simulink model "PMSM_2017b_WithRslvr"  (R2017b)
settings: Solver=FixedStepDiscrete  StartTime=0.0  StopTime=0.2  FixedStep=Ts  RelTol=1e-4  EnableMultiTasking=on
values from neighbouring files (symbols this model uses):
  Ba = 0    [initialization.m]
  Fl = 0.007    [initialization.m]
  flux = Kt/(1.5*P*sqrt(2))    [initialization.m]
  fpwm = 1e4    (= 10000)    [initialization.m]
  Imax = 6*sqrt(2)    [initialization.m]
  J = 9.96e-5    (= 9.96e-05)    [initialization.m]
  K1 = wn^2    (= 1000000)    [initialization.m]
  K2 = 2*fei/wn    (= 0.002)    [initialization.m]
  K_resolver = 1    [initialization.m]
  Ki_Cctrl_d = Rs/(4*Tpwm)    (= 22125)    [initialization.m]
  Ki_Cctrl_q = parameters(4)    [cal_n.m]    (also in draw.m; draw_n_I.m; initialization.m = 1)
  Ki_Spdctrl = parameters(2)    [cal_n.m]    (also in draw.m; draw_n_I.m; initialization.m = 1)
  Kp_Cctrl_d = Ld/(4*Tpwm)    (= 462.5)    [initialization.m]
  Kp_Cctrl_q = parameters(3)    [cal_n.m]    (also in draw.m; draw_n_I.m; initialization.m = 1)
  Kp_Spdctrl = parameters(1)    [cal_n.m]    (also in draw.m; draw_n_I.m; initialization.m = 1)
  Kt = 1.32    [initialization.m]
  Ld = 0.185    [initialization.m]
  Lq = 0.185    [initialization.m]
  P = X    [PSO.m]    (also in initialization.m = 2)
  Rs = 17.7/2    (= 8.85)    [initialization.m]
  SinPeakValue = 0.95104    [initialization.m]
  TestCurrentController = 0    [initialization.m]
  Tf = 0.08    [initialization.m]
  Tpwm = 1e-4    (= 0.0001)    [initialization.m]
  Ts = 1e-5    (= 1e-05)    [initialization.m]
  Udc = 230    [initialization.m]
  UseAgAtan2 = 0    [initialization.m]
  UseAgSim = 1    [initialization.m]
  wm_base = 3000*pi/30    (= 314.159265359)    [initialization.m]
undefined symbols (not defined in the file or in its folder): DiscIntNeverNeededParam
libraries: powerlib x6, simulink x5, dspmtrx3 x1
settings Model: Creator=SUN  LastModifiedBy=Administrator
settings SolverCC: ZeroCrossControl=DisableAll
settings DataIOCC: LimitDataPoints=on  SaveFormat=Array  SignalLoggingSaveFormat=ModelDataLogs
settings OptimizationCC: ExpressionDepthLimit=2147483647  InitFltsAndDblsToZero=on  LifeSpan=inf
settings DebuggingCC: UnderspecifiedInitializationDetection=Classic  MergeDetectMultiDrivingBlocksExec=none  SolverPrmCheckMsg=warning  FcnCallInpInsideContextMsg=warning  StateNameClashWarn=warning  SFUnexpectedBacktrackingDiag=warning  SFNoUnconditionalDefaultTransitionDiag=warning  SFExecutionAtInitializationDiag=none
settings HardwareCC: ProdBitPerPointer=32  ProdBitPerSizeT=32  ProdBitPerPtrDiffT=32  ProdLargestAtomicFloat=None  ProdIntDivRoundTo=Undefined  ProdEndianess=Unspecified  ProdWordSize=32  ProdHWDeviceType=32-bit Generic
settings ModelReferenceCC: PropagateSignalLabelsOutOfModel=off
settings CodeAppCC: StateflowObjectComments=on
settings GRTTargetCC: TargetLangStandard=C89/C90 (ANSI)  GeneratePreprocessorConditionals=Disable all  CombineOutputUpdateFcns=off  GRTInterface=on
settings ConfigComp: CovMetricSettings=dw  CovHtmlReporting=on  CovSaveCumulativeToWorkspaceVar=on  CovSaveSingleToWorkspaceVar=on  CovExternalEMLEnable=off
settings SimscapeCC: SimscapeNormalizeSystem=off

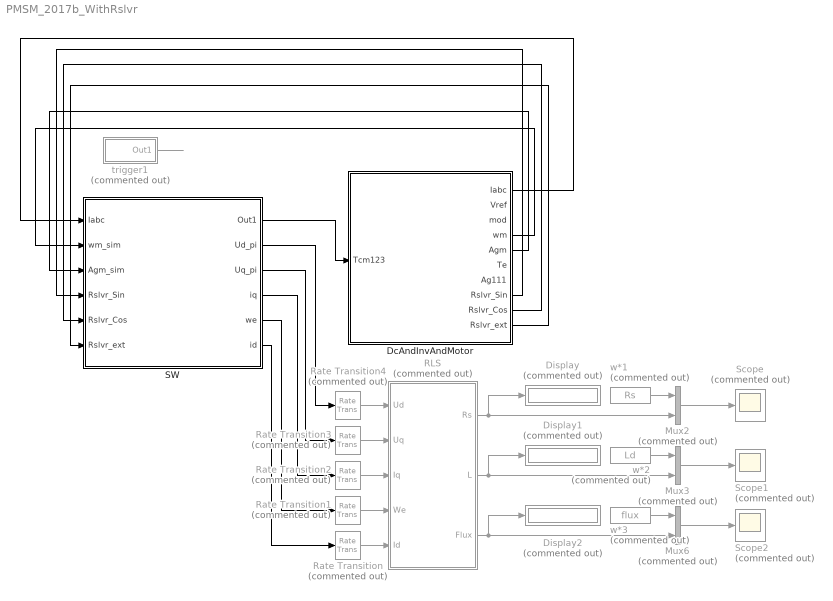
== system PMSM_2017b_WithRslvr ==
  DcAndInvAndMotor : Subsystem
  Display : Display  Commented=on
  Display1 : Display  Commented=on
  Display2 : Display  Commented=on
  Mux2 : Mux  Commented=on  Inputs=2
  Mux3 : Mux  Commented=on  Inputs=2
  Mux6 : Mux  Commented=on  Inputs=2
  RLS : Subsystem  Commented=on
      mask Display: disp('RLS');
  Rate Transition{,1..4} (5 alike) : RateTransition  Commented=on
  SW : Subsystem
  Scope : Scope  Commented=on
  Scope1 : Scope  Commented=on
  Scope2 : Scope  Commented=on
  trigger1 : Subsystem  Commented=on
  w*1 : Constant  Commented=on  Value=Rs
  w*2 : Constant  Commented=on  Value=Ld
  w*3 : Constant  Commented=on  Value=flux
  wires:
  w*3/1 -> Mux6/1
  Mux6/1 -> Scope2/1
  RLS/3(Flux) -> Display2/1, Mux6/2
  w*2/1 -> Mux3/1
  Mux3/1 -> Scope1/1
  w*1/1 -> Mux2/1
  RLS/1(Rs) -> Mux2/2, Display/1
  Mux2/1 -> Scope/1
  RLS/2(L) -> Display1/1, Mux3/2
  trigger1/1(Out1) -> ?
  SW/1(Out1) -> DcAndInvAndMotor/1(Tcm123)
  DcAndInvAndMotor/1(Iabc) -> SW/1(Iabc)
  SW/4(iq) -> Rate Transition2/1
  SW/5(we) -> Rate Transition1/1
  SW/2(Ud_pi) -> Rate Transition4/1
  SW/3(Uq_pi) -> Rate Transition3/1
  SW/6(id) -> Rate Transition/1
  Rate Transition/1 -> RLS/5(Id)
  Rate Transition1/1 -> RLS/4(We)
  Rate Transition2/1 -> RLS/3(Iq)
  Rate Transition3/1 -> RLS/2(Uq)
  Rate Transition4/1 -> RLS/1(Ud)
  DcAndInvAndMotor/5(Agm) -> SW/3(Agm_sim)
  DcAndInvAndMotor/8(Rslvr_Sin) -> SW/4(Rslvr_Sin)
  DcAndInvAndMotor/9(Rslvr_Cos) -> SW/5(Rslvr_Cos)
  DcAndInvAndMotor/10(Rslvr_ext) -> SW/6(Rslvr_ext)
  DcAndInvAndMotor/4(wm) -> SW/2(wm_sim)

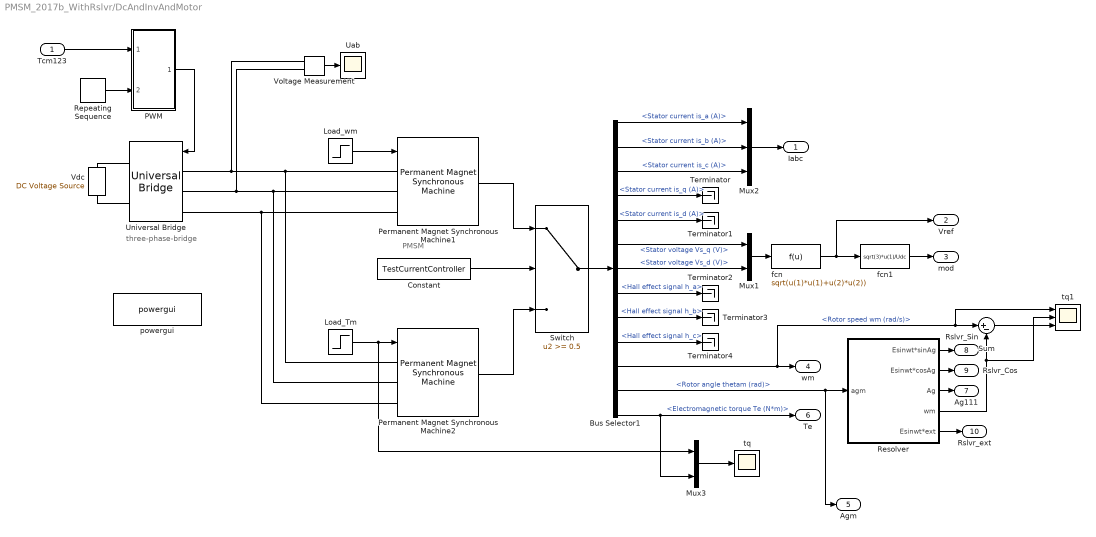
== system PMSM_2017b_WithRslvr/DcAndInvAndMotor ==
  note: three-phase-bridge
  note: PMSM
  Tcm123 : Inport
  Bus Selector1 : BusSelector  OutputSignals=Stator current is_a (A),Stator current is_b (A),Stator current is_c (A),Stator current is_q (A),Stator current is_d (A),Stator voltage Vs_q (V),Stator voltage Vs_d (V),Hall effect signal h_a,Hall effect signal h_b,Hall effect signal h_c,Rotor speed wm (rad/s),Rotor angle thetam (rad),Electromagnetic torque Te (N*m)
  Constant : Constant  Value=TestCurrentController
  Load_Tm : Step  Time=0.15  After=0  SampleTime=0
  Load_wm : Step  Time=0.15  Before=30  After=100  SampleTime=0
  Mux1 : Mux  Inputs=2
  Mux2 : Mux  Inputs=3
  Mux3 : Mux  Inputs=2
  PWM : Subsystem
  Permanent Magnet Synchronous Machine1 : powerlib/Machines/Permanent Magnet Synchronous Machine  NbPhases=3  FluxDistribution=Sinusoidal  RotorType=Salient-pole  MechanicalLoad=Speed w  PresetModel=No  ShowDetailedParameters=on  MeasurementBus=off  Resistance=Rs  Inductance=8.5e-3  dqInductances=[Ld Lq]  La=Lq  MachineConstant=Flux linkage established by magnets (V.s)  Flux=flux  VoltageCst=112.8644  TorqueCst=0.93338  Flat=120  Mechanical=[J Fl P Tf]  PolePairs=P  InitialConditions=[0,0,0,0]  InitialConditions5ph=[0 0 0 0 0 0]  TsPowergui=0  TsBlock=-1  RefAngle=Aligned with phase A axis (original Park)
      settings: SourceProductName=Simscape Power Systems
  Permanent Magnet Synchronous Machine2 : powerlib/Machines/Permanent Magnet Synchronous Machine  NbPhases=3  FluxDistribution=Sinusoidal  RotorType=Salient-pole  MechanicalLoad=Torque Tm  PresetModel=No  ShowDetailedParameters=on  MeasurementBus=off  Resistance=Rs  Inductance=8.5e-3  dqInductances=[Ld Lq]  La=Lq  MachineConstant=Flux linkage established by magnets (V.s)  Flux=flux  VoltageCst=112.8644  TorqueCst=0.93338  Flat=120  Mechanical=[J Fl P Tf]  PolePairs=P  InitialConditions=[0,0,0,0]  InitialConditions5ph=[0 0 0 0 0 0]  TsPowergui=0  TsBlock=-1  RefAngle=Aligned with phase A axis (original Park)
      settings: SourceProductName=Simscape Power Systems
  Repeating Sequence : simulink/Sources/Repeating Sequence  rep_seq_t=[0 Tpwm/2 Tpwm]  rep_seq_y=[0 Tpwm/2 0]
  Resolver : Subsystem
  Sum : Sum  Inputs=|+-
  Switch : Switch  Threshold=0.5
  Terminator{,1..4} (5 alike) : Terminator
  Uab : Scope
  Universal Bridge : powerlib/Power Electronics/Universal Bridge  Arms=3  SnubberResistance=1e5  SnubberCapacitance=inf  Device=IGBT / Diodes  Ron=1e-3  Lon=0  ForwardVoltages="[  0  0  ]"  ForwardVoltage=0  GTOparameters=[ 10e-6 , 20e-6 ]  IGBTparameters=[ 1e-6 , 2e-6 ]  Measurements=None  Measurements_2=None  converterType=Rectifier
  Vdc : powerlib/Electrical Sources/DC Voltage Source  Amplitude=Udc  Measurements=Voltage
  Voltage Measurement : powerlib/Measurements/Voltage Measurement  PhasorSimulation=off  OutputType=Complex  PSBequivalent=0
  fcn : Fcn  Expr=sqrt(u(1)*u(1)+u(2)*u(2))
  fcn1 : Fcn  Expr=sqrt(3)*u(1)/Udc
  powergui : powerlib/powergui  SimulationMode=Discrete  SampleTime=Ts  frequency=60  Iterations=50  frequencyindice=0  Pbase=100e6  ErrMax=1e-4  UnitsV=kV  UnitsW=MW  buscounter=0  FunctionMessages=off  echomessages=off  EnableUseOfTLC=off  CurrentSourceSwitches=off  DisableSnubberDevices=off  DisableRonSwitches=off  DisableVfSwitches=off  DisplayEquations=off  SolverType=Backward Euler  Interpol=off  ExternalGateDelay=off  methode=off  Ts=0  x0status=blocks  SPID=off  SwTol=0  HookPort=off  RestoreLinks=warning  ResistiveCurrentMeasurement=off  Frange=[0:2:500]  Ylog=off  Xlog=on  ShowGrid=off  save=off  variable=ZData  structure=0  ZoomFFT=on  StartTime=0.0  cycles=1  DisplayStyle=1  fundamental=60  FreqAxis=off  MaxFrequency=1000  frequencyindicesteady=1  RmsSteady=1  display=off
  tq : Scope
  tq1 : Scope  NumInputPorts=3
  Iabc : Outport
  Vref : Outport  Port=2
  mod : Outport  Port=3
  wm : Outport  Port=4
  Agm : Outport  Port=5
  Te : Outport  Port=6
  Ag111 : Outport  Port=7
  Rslvr_Sin : Outport  Port=8
  Rslvr_Cos : Outport  Port=9
  Rslvr_ext : Outport  Port=10
  wires:
  Voltage Measurement/1 -> Uab/1
  Mux1/1 -> fcn/1
  fcn1/1 -> mod/1
  fcn/1 -> Vref/1, fcn1/1
  Bus Selector1/1 -> Mux2/1  "<Stator current is_a (A)>"
  Bus Selector1/2 -> Mux2/2  "<Stator current is_b (A)>"
  Bus Selector1/3 -> Mux2/3  "<Stator current is_c (A)>"
  Mux2/1 -> Iabc/1
  Bus Selector1/6 -> Mux1/1  "<Stator voltage Vs_q (V)>"
  Bus Selector1/7 -> Mux1/2  "<Stator voltage Vs_d (V)>"
  Bus Selector1/13 -> Mux3/2, Te/1  "<Electromagnetic torque Te (N*m)>"
  Bus Selector1/11 -> tq1/1, Sum/1, wm/1  "<Rotor speed wm (rad/s)>"
  Bus Selector1/4 -> Terminator/1  "<Stator current is_q (A)>"
  Bus Selector1/5 -> Terminator1/1  "<Stator current is_d (A)>"
  Bus Selector1/8 -> Terminator2/1  "<Hall effect signal h_a>"
  Bus Selector1/9 -> Terminator3/1  "<Hall effect signal h_b>"
  Bus Selector1/10 -> Terminator4/1  "<Hall effect signal h_c>"
  Permanent Magnet Synchronous Machine1/1 -> Switch/1
  Permanent Magnet Synchronous Machine2/1 -> Switch/3
  Switch/1 -> Bus Selector1/1
  Constant/1 -> Switch/2
  Load_wm/1 -> Permanent Magnet Synchronous Machine1/1
  Load_Tm/1 -> Mux3/1, Permanent Magnet Synchronous Machine2/1
  Mux3/1 -> tq/1
  PWM/1(PWM) -> Universal Bridge/1
  Repeating Sequence/1 -> PWM/2(Carrier)
  Tcm123/1 -> PWM/1(Tcm123)
  Bus Selector1/12 -> Agm/1, Resolver/1(agm)  "<Rotor angle thetam (rad)>"
  Resolver/4(wm) -> tq1/2, Sum/2
  Resolver/3(Ag) -> Ag111/1
  Sum/1 -> tq1/3
  Resolver/2(Esinwt*cosAg) -> Rslvr_Cos/1
  Resolver/1(Esinwt*sinAg) -> Rslvr_Sin/1
  Resolver/5(Esinwt*ext) -> Rslvr_ext/1
  connections:
  Universal Bridge/RConn1 -- Vdc/RConn1
  Universal Bridge/RConn2 -- Vdc/LConn1
  Permanent Magnet Synchronous Machine1/LConn1 -- Permanent Magnet Synchronous Machine2/LConn1 -- Voltage Measurement/LConn1 -- Universal Bridge/LConn1
  Permanent Magnet Synchronous Machine1/LConn2 -- Permanent Magnet Synchronous Machine2/LConn2 -- Voltage Measurement/LConn2 -- Universal Bridge/LConn2
  Permanent Magnet Synchronous Machine1/LConn3 -- Permanent Magnet Synchronous Machine2/LConn3 -- Universal Bridge/LConn3

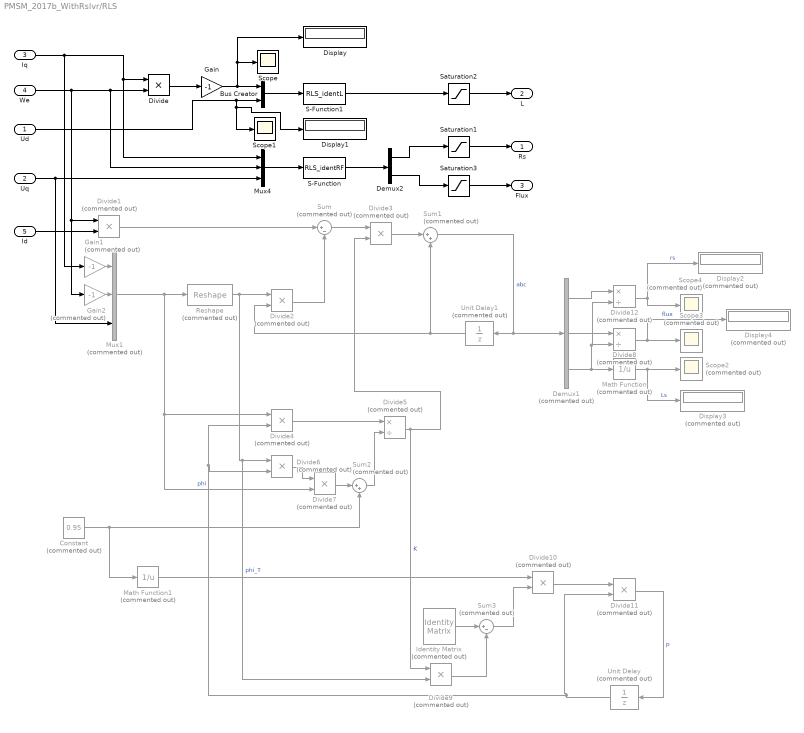
== system PMSM_2017b_WithRslvr/RLS ==
  Ud : Inport
  Uq : Inport  Port=2
  Iq : Inport  Port=3
  We : Inport  Port=4
  Id : Inport  Port=5
  Bus Creator : BusCreator  Inputs=2
  Constant : Constant  Commented=on  Value=0.95
  Demux1 : Demux  Commented=on  Outputs=3
  Demux2 : Demux  Outputs=2
  Display : Display
  Display1 : Display
  Display2 : Display  Commented=on
  Display3 : Display  Commented=on
  Display4 : Display  Commented=on
  Divide : Product  Inputs=**
  Divide{1..4,6..7,9..11} (9 alike) : Product  Commented=on  Inputs=**
  Divide12 : Product  Commented=on  Inputs=*/
  Divide5 : Product  Commented=on  Inputs=*/
  Divide8 : Product  Commented=on  Inputs=*/
  Gain : Gain  Gain=-1
  Gain1 : Gain  Commented=on  Gain=-1
  Gain2 : Gain  Commented=on  Gain=-1
  Identity Matrix : dspmtrx3/Identity Matrix  Commented=on  Inherit=off  N=1  Ts=1  dataType=double  isSigned=on  wordLen=16  udDataType=sfix(16)  fracBitsMode=Best precision  numFracBits=15  OutDataTypeStr=double  LastOutDataTypeStr=double
      settings: SourceProductName=DSP System Toolbox
  Math Function : Math  Commented=on  Operator=reciprocal  SaturateOnIntegerOverflow=on
  Math Function1 : Math  Commented=on  Operator=reciprocal  SaturateOnIntegerOverflow=on
  Mux1 : Mux  Commented=on  Inputs=3
  Mux4 : Mux  Inputs=3
  Reshape : Reshape  Commented=on  OutputDimensionality=Customize  OutputDimensions=[1,3]
  S-Function : S-Function  FunctionName=RLS_identRF  SFunctionDeploymentMode=off  EnableBusSupport=off
  S-Function1 : S-Function  FunctionName=RLS_identL  SFunctionDeploymentMode=off  EnableBusSupport=off
  Saturation1 : Saturate  UpperLimit=25  LowerLimit=0
  Saturation2 : Saturate  UpperLimit=1  LowerLimit=0
  Saturation3 : Saturate  UpperLimit=1  LowerLimit=0
  Scope : Scope
  Scope1 : Scope
  Scope2 : Scope  Commented=on
  Scope3 : Scope  Commented=on
  Scope4 : Scope  Commented=on
  Sum : Sum  Commented=on  Inputs=|+-
  Sum1 : Sum  Commented=on  Inputs=|++
  Sum2 : Sum  Commented=on  Inputs=|++
  Sum3 : Sum  Commented=on  Inputs=|+-
  Unit Delay : UnitDelay  Commented=on  SampleTime=-1
  Unit Delay1 : UnitDelay  Commented=on  InitialCondition=[0.1 0.1 0.1]  SampleTime=-1
  Rs : Outport
  L : Outport  Port=2
  Flux : Outport  Port=3
  wires:
  Divide/1 -> Gain/1
  Gain/1 -> Display/1, Scope/1, Bus Creator/1
  Bus Creator/1 -> S-Function1/1
  S-Function1/1 -> Saturation2/1
  Mux4/1 -> S-Function/1
  S-Function/1 -> Demux2/1
  Demux2/1 -> Saturation1/1
  Iq/1 -> Divide/1, Mux4/1, Gain1/1
  We/1 -> Gain2/1, Divide1/1, Divide/2, Mux4/2
  Ud/1 -> Display1/1, Scope1/1, Bus Creator/2
  Uq/1 -> Mux1/3, Mux4/3
  Saturation3/1 -> Flux/1
  Demux2/2 -> Saturation3/1
  Saturation2/1 -> L/1
  Saturation1/1 -> Rs/1
  Gain1/1 -> Mux1/1
  Gain2/1 -> Mux1/2
  Mux1/1 -> Reshape/1, Divide4/1, Divide7/2  "phi"
  Id/1 -> Divide1/2
  Divide2/1 -> Sum/2
  Sum/1 -> Divide3/1
  Divide5/1 -> Divide9/1, Divide3/2  "K"
  Divide3/1 -> Sum1/1
  Unit Delay1/1 -> Sum1/2, Divide2/2
  Sum1/1 -> Unit Delay1/1, Demux1/1  "abc"
  Reshape/1 -> Divide9/2, Divide6/1, Divide2/1  "phi_T"
  Divide4/1 -> Divide5/1
  Divide6/1 -> Divide7/1
  Divide7/1 -> Sum2/1
  Constant/1 -> Math Function1/1, Sum2/2
  Sum2/1 -> Divide5/2
  Identity Matrix/1 -> Sum3/1
  Divide9/1 -> Sum3/2
  Math Function1/1 -> Divide10/1
  Sum3/1 -> Divide10/2
  Divide10/1 -> Divide11/1
  Divide11/1 -> Unit Delay/1  "p"
  Unit Delay/1 -> Divide11/2, Divide6/2, Divide4/2
  Demux1/3 -> Divide12/2, Divide8/2, Math Function/1
  Math Function/1 -> Display3/1, Scope2/1  "Ls"
  Demux1/2 -> Divide8/1
  Divide8/1 -> Display4/1, Scope3/1  "flux"
  Demux1/1 -> Divide12/1
  Divide12/1 -> Display2/1, Scope4/1  "rs"
  Divide1/1 -> Sum/1

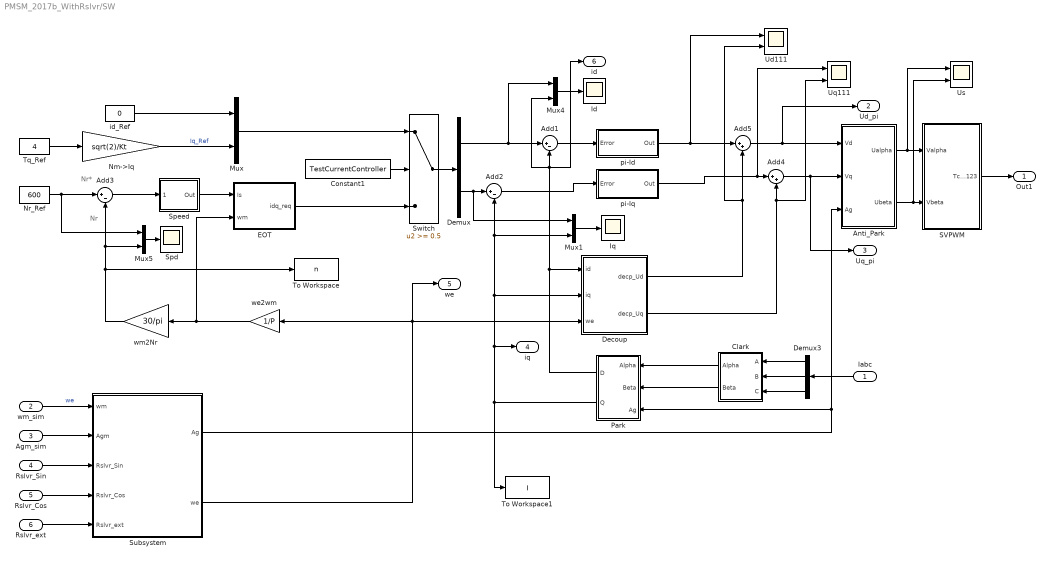
== system PMSM_2017b_WithRslvr/SW ==
  note: Nr*
  note: Nr
  Iabc : Inport
  wm_sim : Inport  Port=2
  Agm_sim : Inport  Port=3
  Rslvr_Sin : Inport  Port=4
  Rslvr_Cos : Inport  Port=5
  Rslvr_ext : Inport  Port=6
  Add1 : Sum  Inputs=|+-
  Add2 : Sum  Inputs=|+-
  Add3 : Sum  Inputs=|+-
  Add4 : Sum  Inputs=|++
  Add5 : Sum  Inputs=|++
  Anti_Park : Subsystem
  Clark : Subsystem
  Constant1 : Constant  Value=TestCurrentController
  Decoup : Subsystem
  Demux : Demux  Outputs=2
  Demux3 : Demux  Outputs=3
  EOT : Subsystem
  Id : Scope
  Iq : Scope
  Mux{,1,4..5} (4 alike) : Mux  Inputs=2
  Nm->Iq : Gain  Gain=sqrt(2)/Kt
  Nr_Ref : Constant  Value=600
  Park : Subsystem
  SVPWM : Subsystem
  Spd : Scope
  Speed : Subsystem  AncestorBlock=|  DialogController=POWERSYS.PowerSysDialog  mask(Discrete PI Controller){Kpw=Kp_Spdctrl, Kiw=Ki_Spdctrl, Ba=Ba, Par_Limits=[Imax -Imax], Init=0, Ts=-1}
      | powerlib_extras/Discrete 
      | Control Blocks/Discrete
      | PI Controller
      mask prompts: Kpw "Proportional gain (Kp):"; Kiw "Integral gain (Ki):"; Ba "feedback gain (Ba)"; Par_Limits "Output limits: [ Upper   Lower ]"; Init "Output initial value:"; Ts "Sample time:"
      mask help: This block implements a discrete PI controller.
      mask init:
      | UpperLimit=Par_Limits(1);
      | LowerLimit=Par_Limits(2);
      | power_initmask();
      mask Help: This block is part of a subset of blocks in the Extras library that does not have documentation associated with it, other than the block mask description.
      mask Display: disp('PI');
  Subsystem : Subsystem
  Switch : Switch  Threshold=0.5
  To Workspace : ToWorkspace  VariableName=n  SaveFormat=Structure With Time  SampleTime=-1
  To Workspace1 : ToWorkspace  VariableName=I  SaveFormat=Structure With Time  SampleTime=-1
  Tq_Ref : Constant  Value=4
  Ud111 : Scope  NumInputPorts=2
  Uq111 : Scope  NumInputPorts=2
  Us : Scope  NumInputPorts=2
  id_Ref : Constant  Value=0
  pi-Id : Subsystem  AncestorBlock=|  DialogController=POWERSYS.PowerSysDialog  mask(Discrete PI Controller){Kp=Kp_Cctrl_d, Ki=Ki_Cctrl_d, Par_Limits=[Udc*sqrt(1/3) -Udc*sqrt(1/3)], Init=0, Ts=-1}
      | powerlib_extras/Discrete 
      | Control Blocks/Discrete
      | PI Controller
      mask prompts: Kp "Proportional gain (Kp):"; Ki "Integral gain (Ki):"; Par_Limits "Output limits: [ Upper   Lower ]"; Init "Output initial value:"; Ts "Sample time:"
      mask help: This block implements a discrete PI controller.
      mask init:
      | UpperLimit=Par_Limits(1);
      | LowerLimit=Par_Limits(2);
      | power_initmask();
      mask Help: This block is part of a subset of blocks in the Extras library that does not have documentation associated with it, other than the block mask description.
      mask Display: disp('PI');
  pi-Iq : Subsystem  AncestorBlock=|  DialogController=POWERSYS.PowerSysDialog  mask(Discrete PI Controller){Kp=Kp_Cctrl_q, Ki=Ki_Cctrl_q, Par_Limits=[Udc*sqrt(1/3) -Udc*sqrt(1/3)], Init=0, Ts=-1}
      | powerlib_extras/Discrete 
      | Control Blocks/Discrete
      | PI Controller
      mask prompts: Kp "Proportional gain (Kp):"; Ki "Integral gain (Ki):"; Par_Limits "Output limits: [ Upper   Lower ]"; Init "Output initial value:"; Ts "Sample time:"
      mask help: This block implements a discrete PI controller.
      mask init:
      | UpperLimit=Par_Limits(1);
      | LowerLimit=Par_Limits(2);
      | power_initmask();
      mask Help: This block is part of a subset of blocks in the Extras library that does not have documentation associated with it, other than the block mask description.
      mask Display: disp('PI');
  we2wm : Gain  Gain=1/P
  wm2Nr : Gain  Gain=30/pi
  Out1 : Outport
  Ud_pi : Outport  Port=2
  Uq_pi : Outport  Port=3
  iq : Outport  Port=4
  we : Outport  Port=5
  id : Outport  Port=6
  wires:
  Add2/1 -> pi-Iq/1(Error)
  Constant1/1 -> Switch/2
  Nr_Ref/1 -> Mux5/1, Add3/1
  Add4/1 -> Uq_pi/1, Anti_Park/2(Vq)
  Decoup/2(decp_Uq) -> Uq111/2, Add4/2
  Park/1(D) -> id/1, Mux4/2, Add1/2, Decoup/1(id)
  SVPWM/1(Tcm123) -> Out1/1
  Add1/1 -> pi-Id/1(Error)
  Mux1/1 -> Iq/1
  EOT/1(idq_req) -> Switch/3
  Add5/1 -> Ud_pi/1, Anti_Park/1(Vd)
  id_Ref/1 -> Mux/1
  Switch/1 -> Demux/1
  Tq_Ref/1 -> Nm->Iq/1
  Mux5/1 -> Spd/1
  Speed/1(Out) -> EOT/1(Is)
  Iabc/1 -> Demux3/1
  we2wm/1 -> EOT/2(wm), wm2Nr/1
  pi-Id/1(Out) -> Ud111/1, Add5/1
  Demux3/2 -> Clark/2(B)
  Decoup/1(decp_Ud) -> Ud111/2, Add5/2
  Demux3/3 -> Clark/3(C)
  Add3/1 -> Speed/1(Error)
  Park/2(Q) -> To Workspace1/1, iq/1, Add2/2, Mux1/2, Decoup/2(iq)
  Demux3/1 -> Clark/1(A)
  Mux/1 -> Switch/1
  wm2Nr/1 -> Mux5/2, Add3/2, To Workspace/1
  pi-Iq/1(Out) -> Uq111/1, Add4/1
  Clark/2(Beta) -> Park/2(Beta)
  Demux/2 -> Mux1/1, Add2/1
  Nm->Iq/1 -> Mux/2  "Iq_Ref"
  Mux4/1 -> Id/1
  Anti_Park/2(Ubeta) -> Us/2, SVPWM/2(Vbeta)
  Demux/1 -> Mux4/1, Add1/1
  Clark/1(Alpha) -> Park/1(Alpha)
  Anti_Park/1(Ualpha) -> Us/1, SVPWM/1(Valpha)
  Agm_sim/1 -> Subsystem/2(Agm)
  Subsystem/2(we) -> we/1, we2wm/1, Decoup/3(we)
  wm_sim/1 -> Subsystem/1(wm)  "we"
  Rslvr_Sin/1 -> Subsystem/3(Rslvr_Sin)
  Rslvr_Cos/1 -> Subsystem/4(Rslvr_Cos)
  Rslvr_ext/1 -> Subsystem/5(Rslvr_ext)
  Subsystem/1(Ag) -> Anti_Park/3(Ag), Park/3(Ag)

== system PMSM_2017b_WithRslvr/trigger1 ==
  Compare To Constant : simulink/Logic and Bit Operations/Compare To Constant  relop=>=  const=Tpwm/Ts  OutDataTypeStr=boolean
  Constant : Constant
  Constant1 : Constant  Value=0
  Delay : Delay  DelayLength=1  InitialCondition=9
  Sum : Sum
  Switch : Switch
  Out1 : Outport
  wires:
  Constant/1 -> Sum/1
  Sum/1 -> Switch/3, Compare To Constant/1
  Delay/1 -> Sum/2
  Compare To Constant/1 -> Out1/1, Switch/2
  Switch/1 -> Delay/1
  Constant1/1 -> Switch/1

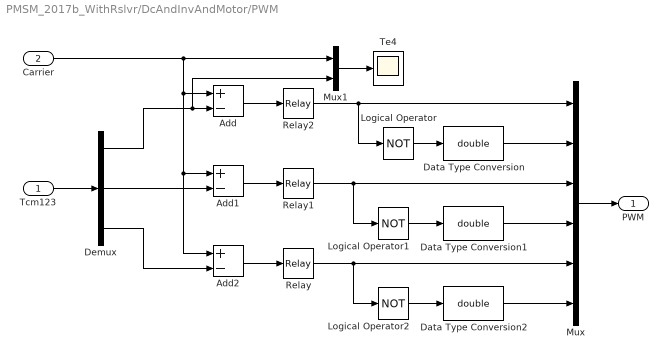
== system PMSM_2017b_WithRslvr/DcAndInvAndMotor/PWM ==
  Tcm123 : Inport
  Carrier : Inport  Port=2
  Add : Sum  Inputs=+-
  Add1 : Sum  Inputs=+-
  Add2 : Sum  Inputs=+-
  Data Type Conversion : DataTypeConversion  OutDataTypeStr=double
  Data Type Conversion1 : DataTypeConversion  OutDataTypeStr=double
  Data Type Conversion2 : DataTypeConversion  OutDataTypeStr=double
  Demux : Demux  Outputs=3
  Logical Operator : Logic  Operator=NOT  AllPortsSameDT=off  OutDataTypeStr=boolean
  Logical Operator1 : Logic  Operator=NOT  AllPortsSameDT=off  OutDataTypeStr=boolean
  Logical Operator2 : Logic  Operator=NOT  AllPortsSameDT=off  OutDataTypeStr=boolean
  Mux : Mux  Inputs=6
  Mux1 : Mux  Inputs=2
  Relay : Relay  OffSwitchValue=-eps
  Relay1 : Relay  OffSwitchValue=-eps
  Relay2 : Relay  OffSwitchValue=-eps
  Te4 : Scope
  PWM : Outport
  wires:
  Demux/3 -> Add2/2
  Demux/2 -> Add1/2
  Demux/1 -> Mux1/2, Add/2
  Relay/1 -> Mux/5, Logical Operator2/1
  Relay1/1 -> Mux/3, Logical Operator1/1
  Mux/1 -> PWM/1
  Data Type Conversion/1 -> Mux/2
  Data Type Conversion1/1 -> Mux/4
  Data Type Conversion2/1 -> Mux/6
  Logical Operator2/1 -> Data Type Conversion2/1
  Logical Operator1/1 -> Data Type Conversion1/1
  Logical Operator/1 -> Data Type Conversion/1
  Add1/1 -> Relay1/1
  Add2/1 -> Relay/1
  Add/1 -> Relay2/1
  Tcm123/1 -> Demux/1
  Mux1/1 -> Te4/1
  Relay2/1 -> Mux/1, Logical Operator/1
  Carrier/1 -> Mux1/1, Add/1, Add2/1, Add1/1

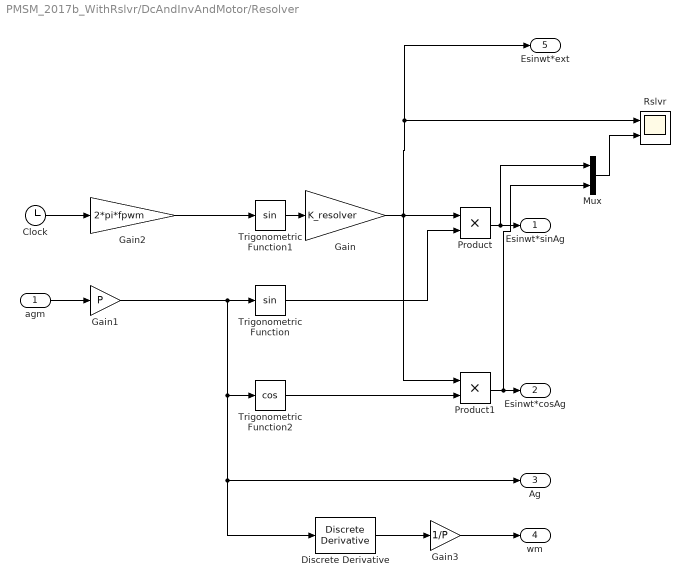
== system PMSM_2017b_WithRslvr/DcAndInvAndMotor/Resolver ==
  agm : Inport
  Clock : Clock
  Discrete Derivative : simulink/Discrete/Discrete Derivative  gainval=1.0  ICPrevScaledInput=0.0  OutMin=[]  OutMax=[]  OutDataType=fixdt(1, 16)  OutScaling=2^-10  DoSatur=off
  Gain : Gain  Gain=K_resolver
  Gain1 : Gain  Gain=P
  Gain2 : Gain  Gain=2*pi*fpwm
  Gain3 : Gain  Gain=1/P
  Mux : Mux  Inputs=2
  Product : Product
  Product1 : Product
  Rslvr : Scope  NumInputPorts=2
  Trigonometric Function : Trigonometry
  Trigonometric Function1 : Trigonometry
  Trigonometric Function2 : Trigonometry  Operator=cos
  Esinwt*sinAg : Outport
  Esinwt*cosAg : Outport  Port=2
  Ag : Outport  Port=3
  wm : Outport  Port=4
  Esinwt*ext : Outport  Port=5
  wires:
  Clock/1 -> Gain2/1
  Trigonometric Function1/1 -> Gain/1
  Gain2/1 -> Trigonometric Function1/1
  Gain/1 -> Esinwt*ext/1, Rslvr/1, Product1/1, Product/1
  Trigonometric Function/1 -> Product/2
  Trigonometric Function2/1 -> Product1/2
  Product1/1 -> Mux/2, Esinwt*cosAg/1
  Gain1/1 -> Trigonometric Function/1, Discrete Derivative/1, Ag/1, Trigonometric Function2/1
  Discrete Derivative/1 -> Gain3/1
  Gain3/1 -> wm/1
  agm/1 -> Gain1/1
  Product/1 -> Mux/1, Esinwt*sinAg/1
  Mux/1 -> Rslvr/2

== system PMSM_2017b_WithRslvr/SW/Anti_Park ==
  Vd : Inport
  Vq : Inport  Port=2
  Ag : Inport  Port=3
  Fcn : Fcn  Expr=u(1)*cos(u(3))-u(2)*sin(u(3))
  Fcn1 : Fcn  Expr=u(1)*sin(u(3))+u(2)*cos(u(3))
  Mux1 : Mux  Inputs=3
  Ualpha : Outport
  Ubeta : Outport  Port=2
  wires:
  Fcn1/1 -> Ubeta/1
  Fcn/1 -> Ualpha/1
  Mux1/1 -> Fcn/1, Fcn1/1
  Vd/1 -> Mux1/1
  Vq/1 -> Mux1/2
  Ag/1 -> Mux1/3

== system PMSM_2017b_WithRslvr/SW/Clark ==
  A : Inport
  B : Inport  Port=2
  C : Inport  Port=3
  Mux : Mux  Inputs=3
  alpha : Fcn  Expr=(u(1)-0.5*(u(2)+u(3)))*2/3
  beta : Fcn  Expr=sqrt(3)/2*(u(2)-u(3))*2/3
  Alpha : Outport
  Beta : Outport  Port=2
  wires:
  alpha/1 -> Alpha/1
  B/1 -> Mux/2
  C/1 -> Mux/3
  A/1 -> Mux/1
  Mux/1 -> beta/1, alpha/1
  beta/1 -> Beta/1

== system PMSM_2017b_WithRslvr/SW/Decoup ==
  id : Inport
  iq : Inport  Port=2
  we : Inport  Port=3
  Fcn : Fcn  Expr=(u(1)*u(2)*Ld)+(u(2)*flux)
  Fcn1 : Fcn  Expr=-u(1)*u(2)*Lq
  Mux1 : Mux  Inputs=2
  Mux2 : Mux  Inputs=2
  decp_Ud : Outport
  decp_Uq : Outport  Port=2
  wires:
  we/1 -> Mux1/2, Mux2/2
  Mux2/1 -> Fcn/1
  Mux1/1 -> Fcn1/1
  id/1 -> Mux2/1
  iq/1 -> Mux1/1
  Fcn/1 -> decp_Uq/1
  Fcn1/1 -> decp_Ud/1

== system PMSM_2017b_WithRslvr/SW/EOT ==
  Is : Inport
  wm : Inport  Port=2
  Constant : Constant  Value=wm_base
  Constant1 : Constant  Value=0
  Fcn : Fcn  Expr=-u(1)*sqrt(1-(wm_base/u(2))^2)
  Fcn1 : Fcn  Expr=u(1)*(wm_base/u(2))
  Mux : Mux  Inputs=2
  Mux1 : Mux  Inputs=2
  Mux2 : Mux  Inputs=2
  Relational Operator : RelationalOperator  Operator=<=  OutDataTypeStr=boolean  RndMeth=Nearest
  Switch : Switch  Criteria=u2 ~= 0
  idq_req : Outport
  wires:
  Is/1 -> Mux2/1, Mux/2
  wm/1 -> Mux2/2, Relational Operator/1
  Constant/1 -> Relational Operator/2
  Relational Operator/1 -> Switch/2
  Constant1/1 -> Mux/1
  Mux/1 -> Switch/1
  Mux2/1 -> Fcn1/1, Fcn/1
  Fcn/1 -> Mux1/1
  Fcn1/1 -> Mux1/2
  Mux1/1 -> Switch/3
  Switch/1 -> idq_req/1

== system PMSM_2017b_WithRslvr/SW/Park ==
  Alpha : Inport
  Beta : Inport  Port=2
  Ag : Inport  Port=3
  Mux : Mux  Inputs=3
  d : Fcn  Expr=u(1)*cos(u(3))+u(2)*sin(u(3))
  q : Fcn  Expr=-u(1)*sin(u(3))+u(2)*cos(u(3))
  D : Outport
  Q : Outport  Port=2
  wires:
  d/1 -> D/1
  Beta/1 -> Mux/2
  Alpha/1 -> Mux/1
  Mux/1 -> q/1, d/1
  q/1 -> Q/1
  Ag/1 -> Mux/3

== system PMSM_2017b_WithRslvr/SW/SVPWM ==
  Valpha : Inport
  Vbeta : Inport  Port=2
  Sector Caculate : Subsystem
  T1T1 Caculate : Subsystem
  Tcm Caculate : Subsystem
  Tpwm : Constant  Value=Tpwm
  Udc : Constant  Value=Udc
  XYZ Caculate : Subsystem
  Tcm123 : Outport
  wires:
  Vbeta/1 -> XYZ Caculate/2(Ubeta), Sector Caculate/2(Ubeta)
  T1T1 Caculate/1(T1) -> Tcm Caculate/2(T1)
  Valpha/1 -> XYZ Caculate/1(Ualpha), Sector Caculate/1(Ualpha)
  T1T1 Caculate/2(T2) -> Tcm Caculate/3(T2)
  Sector Caculate/1("N ") -> Tcm Caculate/1(N), T1T1 Caculate/1(N)
  XYZ Caculate/1(XYZ) -> T1T1 Caculate/2(XYZ)
  Tpwm/1 -> XYZ Caculate/3(Ts), Tcm Caculate/4(Tpwm), T1T1 Caculate/3(Tpwm)
  Udc/1 -> XYZ Caculate/4(Udc)
  Tcm Caculate/1(Tcm1 Tcm2 Tcm3) -> Tcm123/1

== system PMSM_2017b_WithRslvr/SW/Speed ==
  note: Discrete PID Controller
  Error : Inport  SampleTime=Ts
  Discrete-Time Integrator : DiscreteIntegrator  IntegratorMethod=Integration: Backward Euler  InitialCondition=Init  SampleTime=-1  LimitOutput=on  UpperSaturationLimit=UpperLimit  LowerSaturationLimit=LowerLimit  ICPrevOutput=DiscIntNeverNeededParam  ICPrevScaledInput=DiscIntNeverNeededParam
  Kp1 : Gain  Gain=Ba  SaturateOnIntegerOverflow=on  OutDataTypeStr=Inherit: Same as input  ParamDataTypeStr=Inherit: Same as input
  Kp4 : Gain  Gain=Kpw  SampleTime=Ts  SaturateOnIntegerOverflow=on  OutDataTypeStr=Inherit: Same as input  ParamDataTypeStr=Inherit: Same as input
  Kp5 : Gain  Gain=Kiw  SampleTime=Ts  SaturateOnIntegerOverflow=on  OutDataTypeStr=Inherit: Same as input  ParamDataTypeStr=Inherit: Same as input
  Saturation2 : Saturate  UpperLimit=UpperLimit  LowerLimit=LowerLimit  SampleTime=Ts
  Scope : Scope
  Sum6 : Sum  Inputs=++-  SampleTime=Ts  SaturateOnIntegerOverflow=on  InputSameDT=on  OutDataTypeStr=Inherit: Same as first input
  Zero-Order Hold : ZeroOrderHold  SampleTime=-1
  Out : Outport  SampleTime=Ts  InitialOutput=0
  wires:
  Error/1 -> Kp4/1, Kp5/1
  Zero-Order Hold/1 -> Scope/1, Sum6/1
  Saturation2/1 -> Out/1
  Discrete-Time Integrator/1 -> Sum6/2
  Kp4/1 -> Zero-Order Hold/1
  Sum6/1 -> Saturation2/1
  Kp1/1 -> Sum6/3
  [Nr] -> Kp1/1
  Kp5/1 -> Discrete-Time Integrator/1

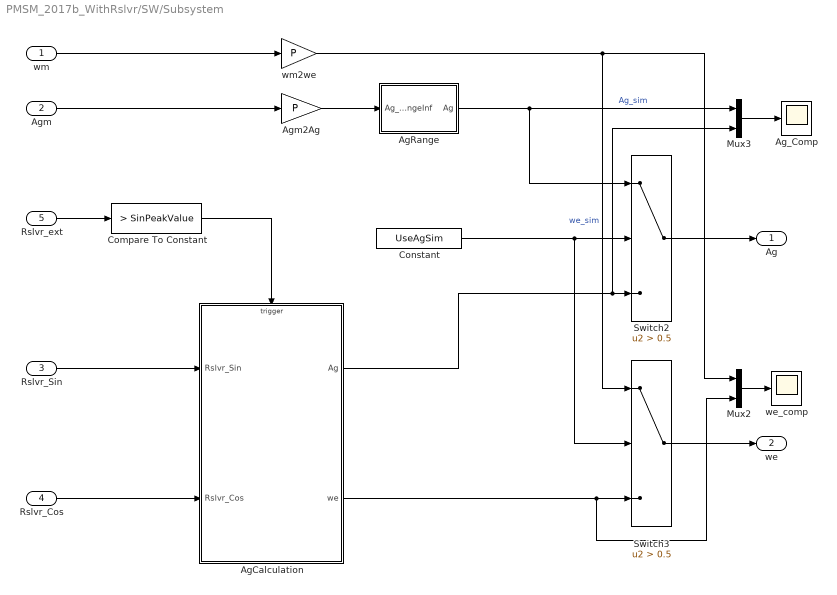
== system PMSM_2017b_WithRslvr/SW/Subsystem ==
  wm : Inport
  Agm : Inport  Port=2
  Rslvr_Sin : Inport  Port=3
  Rslvr_Cos : Inport  Port=4
  Rslvr_ext : Inport  Port=5
  AgCalculation : Subsystem
  AgRange : Subsystem
  Ag_Comp : Scope
  Agm2Ag : Gain  Gain=P
  Compare To Constant : simulink/Logic and Bit Operations/Compare To Constant  relop=>  const=SinPeakValue  OutDataTypeStr=boolean
  Constant : Constant  Value=UseAgSim
  Mux2 : Mux  Inputs=2
  Mux3 : Mux  Inputs=2
  Switch2 : Switch  Criteria=u2 > Threshold  Threshold=0.5
  Switch3 : Switch  Criteria=u2 > Threshold  Threshold=0.5
  we_comp : Scope
  wm2we : Gain  Gain=P
  Ag : Outport
  we : Outport  Port=2
  wires:
  Rslvr_Sin/1 -> AgCalculation/1(Rslvr_Sin)
  Rslvr_Cos/1 -> AgCalculation/2(Rslvr_Cos)
  Rslvr_ext/1 -> Compare To Constant/1
  Compare To Constant/1 -> AgCalculation/Trigger
  wm/1 -> wm2we/1
  Agm/1 -> Agm2Ag/1
  Agm2Ag/1 -> AgRange/1(Ag_RangeInf)
  Switch2/1 -> Ag/1
  AgCalculation/1(Ag) -> Mux3/2, Switch2/3
  AgCalculation/2(we) -> Mux2/2, Switch3/3
  Constant/1 -> Switch3/2, Switch2/2
  Switch3/1 -> we/1
  wm2we/1 -> Switch3/1, Mux2/1  "we_sim"
  Mux2/1 -> we_comp/1
  AgRange/1(Ag) -> Mux3/1, Switch2/1  "Ag_sim"
  Mux3/1 -> Ag_Comp/1

== system PMSM_2017b_WithRslvr/SW/pi-Id ==
  note: Discrete PID Controller
  Error : Inport  SampleTime=Ts
  Discrete-Time Integrator : DiscreteIntegrator  InitialCondition=Init  SampleTime=-1  LimitOutput=on  UpperSaturationLimit=UpperLimit  LowerSaturationLimit=LowerLimit  ICPrevOutput=DiscIntNeverNeededParam  ICPrevScaledInput=DiscIntNeverNeededParam
  Kp4 : Gain  Gain=Kp  SampleTime=Ts  SaturateOnIntegerOverflow=on  OutDataTypeStr=Inherit: Same as input  ParamDataTypeStr=Inherit: Same as input
  Kp5 : Gain  Gain=Ki  SampleTime=Ts  SaturateOnIntegerOverflow=on  OutDataTypeStr=Inherit: Same as input  ParamDataTypeStr=Inherit: Same as input
  Saturation2 : Saturate  UpperLimit=UpperLimit  LowerLimit=LowerLimit  SampleTime=Ts
  Sum6 : Sum  SampleTime=Ts  SaturateOnIntegerOverflow=on  InputSameDT=on  OutDataTypeStr=Inherit: Same as first input
  Zero-Order Hold : ZeroOrderHold  SampleTime=-1
  Out : Outport  SampleTime=Ts  InitialOutput=0
  wires:
  Zero-Order Hold/1 -> Sum6/1
  Saturation2/1 -> Out/1
  Discrete-Time Integrator/1 -> Sum6/2
  Kp4/1 -> Zero-Order Hold/1
  Sum6/1 -> Saturation2/1
  Error/1 -> Kp5/1, Kp4/1
  Kp5/1 -> Discrete-Time Integrator/1

== system PMSM_2017b_WithRslvr/SW/pi-Iq ==
  note: Discrete PID Controller
  Error : Inport  SampleTime=Ts
  Discrete-Time Integrator : DiscreteIntegrator  InitialCondition=Init  SampleTime=-1  LimitOutput=on  UpperSaturationLimit=UpperLimit  LowerSaturationLimit=LowerLimit  ICPrevOutput=DiscIntNeverNeededParam  ICPrevScaledInput=DiscIntNeverNeededParam
  Kp4 : Gain  Gain=Kp  SampleTime=Ts  SaturateOnIntegerOverflow=on  OutDataTypeStr=Inherit: Same as input  ParamDataTypeStr=Inherit: Same as input
  Kp5 : Gain  Gain=Ki  SampleTime=Ts  SaturateOnIntegerOverflow=on  OutDataTypeStr=Inherit: Same as input  ParamDataTypeStr=Inherit: Same as input
  Saturation2 : Saturate  UpperLimit=UpperLimit  LowerLimit=LowerLimit  SampleTime=Ts
  Sum6 : Sum  SampleTime=Ts  SaturateOnIntegerOverflow=on  InputSameDT=on  OutDataTypeStr=Inherit: Same as first input
  Zero-Order Hold : ZeroOrderHold  SampleTime=-1
  Out : Outport  SampleTime=Ts  InitialOutput=0
  wires:
  Zero-Order Hold/1 -> Sum6/1
  Saturation2/1 -> Out/1
  Discrete-Time Integrator/1 -> Sum6/2
  Kp4/1 -> Zero-Order Hold/1
  Sum6/1 -> Saturation2/1
  Error/1 -> Kp5/1, Kp4/1
  Kp5/1 -> Discrete-Time Integrator/1

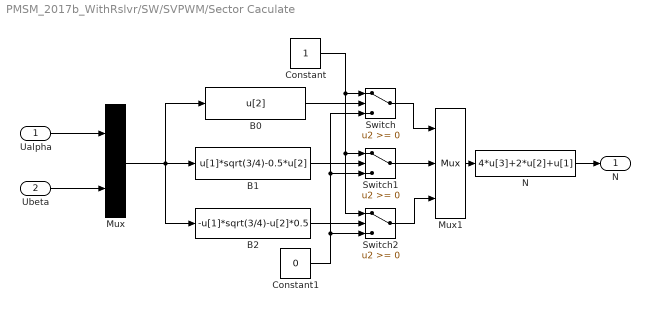
== system PMSM_2017b_WithRslvr/SW/SVPWM/Sector Caculate ==
  Ualpha : Inport
  Ubeta : Inport  Port=2
  B0 : Fcn  Expr=u[2]
  B1 : Fcn  Expr=u[1]*sqrt(3/4)-0.5*u[2]
  B2 : Fcn  Expr=-u[1]*sqrt(3/4)-u[2]*0.5
  Constant : Constant
  Constant1 : Constant  Value=0
  Mux : Mux  Inputs=2
  Mux1 : Mux  Inputs=3
  N : Fcn  Expr=4*u[3]+2*u[2]+u[1]
  Switch : Switch
  Switch1 : Switch
  Switch2 : Switch
  "N " : Outport
  wires:
  Switch2/1 -> Mux1/3
  Switch/1 -> Mux1/1
  Ualpha/1 -> Mux/1
  Ubeta/1 -> Mux/2
  Mux/1 -> B2/1, B1/1, B0/1
  B0/1 -> Switch/2
  B1/1 -> Switch1/2
  B2/1 -> Switch2/2
  Constant/1 -> Switch/1, Switch2/1, Switch1/1
  Constant1/1 -> Switch/3, Switch1/3, Switch2/3
  Switch1/1 -> Mux1/2
  Mux1/1 -> N/1
  N/1 -> "N "/1

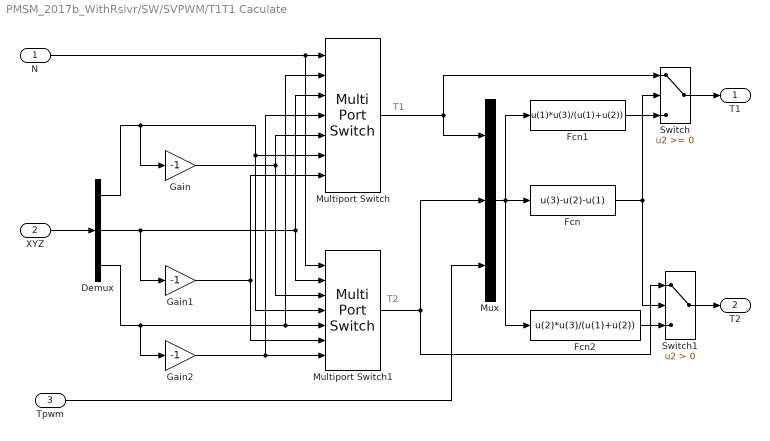
== system PMSM_2017b_WithRslvr/SW/SVPWM/T1T1 Caculate ==
  note: T1
  note: T2
  N : Inport
  XYZ : Inport  Port=2
  Tpwm : Inport  Port=3
  Demux : Demux  Outputs=3
  Fcn : Fcn  Expr=u(3)-u(2)-u(1)
  Fcn1 : Fcn  Expr=u(1)*u(3)/(u(1)+u(2))
  Fcn2 : Fcn  Expr=u(2)*u(3)/(u(1)+u(2))
  Gain : Gain  Gain=-1
  Gain1 : Gain  Gain=-1
  Gain2 : Gain  Gain=-1
  Multiport Switch : MultiPortSwitch  Inputs=6
  Multiport Switch1 : MultiPortSwitch  Inputs=6
  Mux : Mux  Inputs=3
  Switch : Switch
  Switch1 : Switch  Criteria=u2 > Threshold
  T1 : Outport
  T2 : Outport  Port=2
  wires:
  Tpwm/1 -> Mux/3
  XYZ/1 -> Demux/1
  Switch1/1 -> T2/1
  Switch/1 -> T1/1
  Fcn2/1 -> Switch1/3
  Fcn1/1 -> Switch/3
  Fcn/1 -> Switch/2, Switch1/2
  Mux/1 -> Fcn1/1, Fcn/1, Fcn2/1
  Multiport Switch/1 -> Switch/1, Mux/1
  Multiport Switch1/1 -> Switch1/1, Mux/2
  N/1 -> Multiport Switch/1, Multiport Switch1/1
  Demux/2 -> Multiport Switch/3, Multiport Switch1/2, Gain1/1
  Demux/3 -> Multiport Switch1/5, Multiport Switch/2, Gain2/1
  Demux/1 -> Multiport Switch/6, Multiport Switch1/4, Gain/1
  Gain/1 -> Multiport Switch1/3, Multiport Switch/5
  Gain2/1 -> Multiport Switch/4, Multiport Switch1/7
  Gain1/1 -> Multiport Switch1/6, Multiport Switch/7

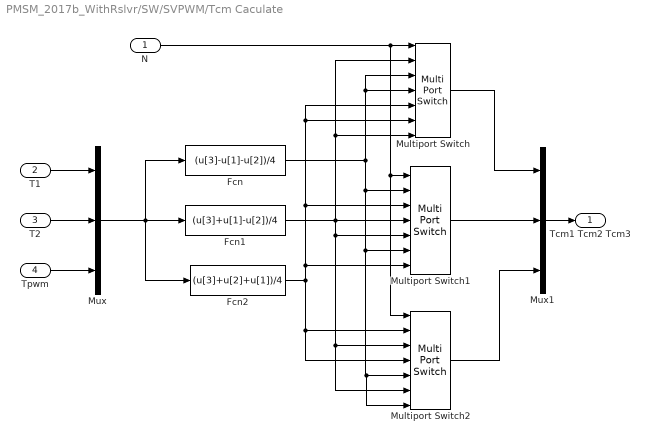
== system PMSM_2017b_WithRslvr/SW/SVPWM/Tcm Caculate ==
  N : Inport
  T1 : Inport  Port=2
  T2 : Inport  Port=3
  Tpwm : Inport  Port=4
  Fcn : Fcn  Expr=(u[3]-u[1]-u[2])/4
  Fcn1 : Fcn  Expr=(u[3]+u[1]-u[2])/4
  Fcn2 : Fcn  Expr=(u[3]+u[2]+u[1])/4
  Multiport Switch : MultiPortSwitch  Inputs=6
  Multiport Switch1 : MultiPortSwitch  Inputs=6
  Multiport Switch2 : MultiPortSwitch  Inputs=6
  Mux : Mux  Inputs=3
  Mux1 : Mux  Inputs=3
  Tcm1 Tcm2 Tcm3 : Outport
  wires:
  Mux/1 -> Fcn2/1, Fcn/1, Fcn1/1
  Tpwm/1 -> Mux/3
  T2/1 -> Mux/2
  T1/1 -> Mux/1
  Multiport Switch2/1 -> Mux1/3
  Multiport Switch1/1 -> Mux1/2
  Multiport Switch/1 -> Mux1/1
  Mux1/1 -> Tcm1 Tcm2 Tcm3/1
  Fcn/1 -> Multiport Switch/3, Multiport Switch/4, Multiport Switch1/6, Multiport Switch2/5, Multiport Switch2/7, Multiport Switch1/2
  Fcn1/1 -> Multiport Switch1/5, Multiport Switch2/3, Multiport Switch2/6, Multiport Switch1/4, Multiport Switch/7, Multiport Switch/2
  Fcn2/1 -> Multiport Switch/5, Multiport Switch/6, Multiport Switch1/3, Multiport Switch1/7, Multiport Switch2/2, Multiport Switch2/4
  N/1 -> Multiport Switch2/1, Multiport Switch1/1, Multiport Switch/1

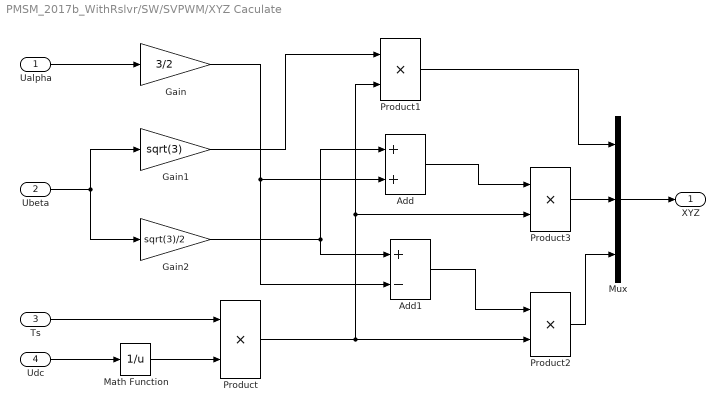
== system PMSM_2017b_WithRslvr/SW/SVPWM/XYZ Caculate ==
  Ualpha : Inport
  Ubeta : Inport  Port=2
  Ts : Inport  Port=3
  Udc : Inport  Port=4
  Add : Sum
  Add1 : Sum  Inputs=+-
  Gain : Gain  Gain=3/2
  Gain1 : Gain  Gain=sqrt(3)
  Gain2 : Gain  Gain=sqrt(3)/2
  Math Function : Math  Operator=reciprocal  SaturateOnIntegerOverflow=on
  Mux : Mux  Inputs=3
  Product{,1..3} (4 alike) : Product  RndMeth=Zero
  XYZ : Outport
  wires:
  Mux/1 -> XYZ/1
  Product1/1 -> Mux/1
  Product3/1 -> Mux/2
  Product2/1 -> Mux/3
  Ualpha/1 -> Gain/1
  Ubeta/1 -> Gain2/1, Gain1/1
  Udc/1 -> Math Function/1
  Math Function/1 -> Product/2
  Ts/1 -> Product/1
  Gain1/1 -> Product1/1
  Product/1 -> Product2/2, Product1/2, Product3/2
  Gain/1 -> Add1/2, Add/2
  Gain2/1 -> Add/1, Add1/1
  Add1/1 -> Product2/1
  Add/1 -> Product3/1

== system PMSM_2017b_WithRslvr/SW/Subsystem/AgCalculation ==
  Rslvr_Sin : Inport
  Rslvr_Cos : Inport  Port=2
  Trigger : TriggerPort  VariantControl=Variant  PortDimensions=1
  Ag_PIcontroller : Subsystem
  Ag_atan2 : Subsystem
  Constant : Constant  Value=UseAgAtan2
  Switch1 : Switch  Criteria=u2 > Threshold  Threshold=0.5
  Switch3 : Switch  Criteria=u2 > Threshold  Threshold=0.5
  Ag : Outport
  we : Outport  Port=2
  wires:
  Rslvr_Sin/1 -> Ag_PIcontroller/1(In1), Ag_atan2/1(In1)
  Rslvr_Cos/1 -> Ag_PIcontroller/2(In2), Ag_atan2/2(In2)
  Ag_PIcontroller/1(Ag) -> Switch3/3
  Ag_atan2/1(Ag) -> Switch3/1
  Switch3/1 -> Ag/1
  Ag_PIcontroller/2(we) -> Switch1/3
  Ag_atan2/2(we) -> Switch1/1
  Switch1/1 -> we/1
  Constant/1 -> Switch1/2, Switch3/2

== system PMSM_2017b_WithRslvr/SW/Subsystem/AgRange ==
  note: To make the Ag is in the range of [-pi,pi]
  Ag_RangeInf : Inport
  Constant : Constant  Value=pi
  Constant2 : Constant  Value=2*pi
  Mod : Math  Operator=mod  SaturateOnIntegerOverflow=on
  Relational Operator : RelationalOperator  OutDataTypeStr=boolean  RndMeth=Simplest
  Sum : Sum  Inputs=|+-
  Switch2 : Switch  Criteria=u2 > Threshold  Threshold=0.5
  Ag : Outport
  wires:
  Sum/1 -> Switch2/1
  Relational Operator/1 -> Switch2/2
  Ag_RangeInf/1 -> Mod/1
  Constant/1 -> Relational Operator/2
  Constant2/1 -> Sum/2, Mod/2
  Mod/1 -> Sum/1, Switch2/3, Relational Operator/1
  Switch2/1 -> Ag/1

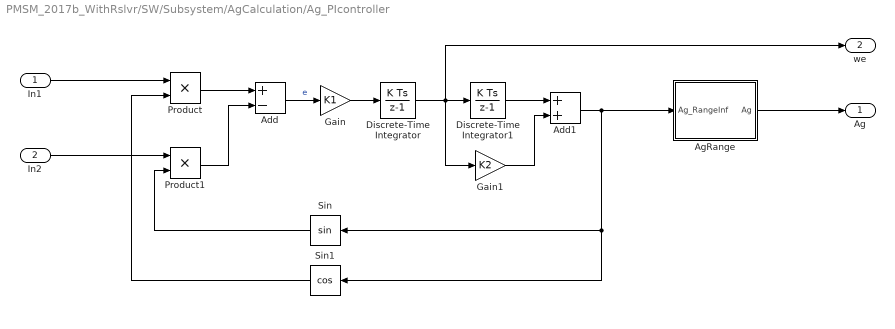
== system PMSM_2017b_WithRslvr/SW/Subsystem/AgCalculation/Ag_PIcontroller ==
  In1 : Inport
  In2 : Inport  Port=2
  Add : Sum  Inputs=+-
  Add1 : Sum
  AgRange : Subsystem
  Discrete-Time Integrator : DiscreteIntegrator  SampleTime=-1  ICPrevOutput=DiscIntNeverNeededParam  ICPrevScaledInput=DiscIntNeverNeededParam
  Discrete-Time Integrator1 : DiscreteIntegrator  SampleTime=-1  ICPrevOutput=DiscIntNeverNeededParam  ICPrevScaledInput=DiscIntNeverNeededParam
  Gain : Gain  Gain=K1
  Gain1 : Gain  Gain=K2
  Product : Product
  Product1 : Product
  Sin : Trigonometry
  Sin1 : Trigonometry  Operator=cos
  Ag : Outport
  we : Outport  Port=2
  wires:
  In2/1 -> Product1/1
  Gain/1 -> Discrete-Time Integrator/1
  Discrete-Time Integrator/1 -> we/1, Gain1/1, Discrete-Time Integrator1/1
  Gain1/1 -> Add1/2
  Discrete-Time Integrator1/1 -> Add1/1
  Product1/1 -> Add/2
  Sin1/1 -> Product/2
  Sin/1 -> Product1/2
  AgRange/1(Ag) -> Ag/1
  Add1/1 -> AgRange/1(Ag_RangeInf), Sin1/1, Sin/1
  Add/1 -> Gain/1  "e"
  Product/1 -> Add/1
  In1/1 -> Product/1

== system PMSM_2017b_WithRslvr/SW/Subsystem/AgCalculation/Ag_atan2 ==
  In1 : Inport
  In2 : Inport  Port=2
  Discrete Derivative : simulink/Discrete/Discrete Derivative  gainval=1.0  ICPrevScaledInput=0.0  OutMin=[]  OutMax=[]  OutDataType=fixdt(1, 16)  OutScaling=2^-10  DoSatur=off
  Sin1 : Trigonometry  Operator=atan2
  Ag : Outport
  we : Outport  Port=2
  wires:
  In1/1 -> Sin1/1
  Sin1/1 -> Ag/1, Discrete Derivative/1
  Discrete Derivative/1 -> we/1
  In2/1 -> Sin1/2

== system PMSM_2017b_WithRslvr/SW/Subsystem/AgCalculation/Ag_PIcontroller/AgRange ==
  note: To make the Ag is in the range of [-pi,pi]
  Ag_RangeInf : Inport
  Constant : Constant  Value=pi
  Constant2 : Constant  Value=2*pi
  Mod : Math  Operator=mod  SaturateOnIntegerOverflow=on
  Relational Operator : RelationalOperator  OutDataTypeStr=boolean  RndMeth=Simplest
  Sum : Sum  Inputs=|+-
  Switch2 : Switch  Criteria=u2 > Threshold  Threshold=0.5
  Ag : Outport
  wires:
  Sum/1 -> Switch2/1
  Relational Operator/1 -> Switch2/2
  Ag_RangeInf/1 -> Mod/1
  Constant/1 -> Relational Operator/2
  Constant2/1 -> Sum/2, Mod/2
  Mod/1 -> Sum/1, Switch2/3, Relational Operator/1
  Switch2/1 -> Ag/1
